simulink model "ThreeMotorModelSimulationXwithRangles"  (R2020b)
settings: Solver=ode14x  StartTime=0.0  StopTime=SimTime  FixedStep=SimStepTime  RelTol=1e-3
InitFcn:
  | StartupScript
StartFcn:
  | StartupScript
values from neighbouring files (symbols this model uses):
  CF = 372.0    (= 372)    [StartupScript.m]
  d2r = pi/180    (= 0.0174532925199)    [StartupScript.m]
  Isat = 10.0    (= 10)    [StartupScript.m]
  Ka = 1    [StartupScript.m]
  Kb = 1    [StartupScript.m]
  Kda = 50    [StartupScript.m]
  Kdb = 280    [StartupScript.m]
  Kdr = 3.4    [StartupScript.m]
  Kia = 150    [StartupScript.m]
  Kib = 200    [StartupScript.m]
  Kir = 6.1    [StartupScript.m]
  Kma = 19.5*1e-3    (= 0.0195)    [StartupScript.m]
  Kmb = 23.4*1e-3    (= 0.0234)    [StartupScript.m]
  Kmr = 29.9*1e-3    (= 0.0299)    [StartupScript.m]
  Kpa = 1250    [StartupScript.m]
  Kpb = 1500    [StartupScript.m]
  Kpr = 40    [StartupScript.m]
  Kr = 1    [StartupScript.m]
  PidLim = 1024    [StartupScript.m]
  PidUCGain = 5/1024    (= 0.0048828125)    [StartupScript.m]
  r2d = 180/pi    (= 57.2957795131)    [StartupScript.m]
  sensorGain = 1/1024.0    (= 0.0009765625)    [StartupScript.m]
  SimStepTime = 1e-3    (= 0.001)    [StartupScript.m]
  Vsat = 24.0    (= 24)    [StartupScript.m]
libraries: cstblocks x9, simulink x1
settings Model: Creator=nisch  LastModifiedBy=nisch

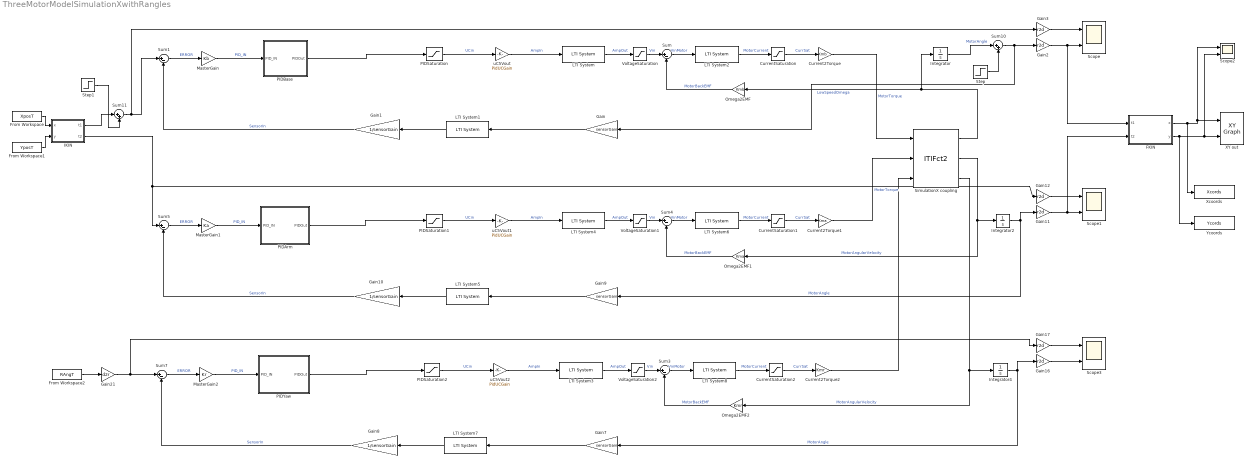
== system ThreeMotorModelSimulationXwithRangles ==
  Current2Torque : Gain  Gain=Kmb
  Current2Torque1 : Gain  Gain=Kma
  Current2Torque2 : Gain  Gain=Kmr
  CurrentSaturation : Saturate  UpperLimit=Isat  LowerLimit=-Isat
  CurrentSaturation1 : Saturate  UpperLimit=Isat  LowerLimit=-Isat
  CurrentSaturation2 : Saturate  UpperLimit=Isat  LowerLimit=-Isat
  FKIN : MATLAB Function  TreatAsAtomicUnit=on
  From Workspace : FromWorkspace  VariableName=XposT
  From Workspace1 : FromWorkspace  VariableName=YposT
  From Workspace2 : FromWorkspace  VariableName=RAngT  SampleTime=-1
  Gain : Gain  Gain=sensorGain
  Gain1 : Gain  Gain=1/sensorGain
  Gain10 : Gain  Gain=1/sensorGain
  Gain{2..3,11..12,16..17} (6 alike) : Gain  Gain=r2d
  Gain21 : Gain  Gain=d2r
  Gain7 : Gain  Gain=sensorGain
  Gain8 : Gain  Gain=1/sensorGain
  Gain9 : Gain  Gain=sensorGain
  IKIN : MATLAB Function  TreatAsAtomicUnit=on
  Integrator : Integrator
  Integrator2 : Integrator
  Integrator4 : Integrator
  LTI System : cstblocks/LTI System  sys=VoltageAmplifier  IC=[]
  LTI System1 : cstblocks/LTI System  sys=Hs  IC=[]
  LTI System2 : cstblocks/LTI System  sys=Electricalb  IC=[]
  LTI System3 : cstblocks/LTI System  sys=VoltageAmplifier  IC=[]
  LTI System4 : cstblocks/LTI System  sys=VoltageAmplifier  IC=[]
  LTI System5 : cstblocks/LTI System  sys=Hs  IC=[]
  LTI System6 : cstblocks/LTI System  sys=Electricala  IC=[]
  LTI System7 : cstblocks/LTI System  sys=Hs  IC=[]
  LTI System8 : cstblocks/LTI System  sys=Electricalr  IC=[]
  MasterGain : Gain  Gain=Kb
  MasterGain1 : Gain  Gain=Ka
  MasterGain2 : Gain  Gain=Kr
  Omega2EMF : Gain  Gain=Kmb
  Omega2EMF1 : Gain  Gain=Kma
  Omega2EMF2 : Gain  Gain=Kmr
  PIDArm : Subsystem
      mask Display: image('MATLABFcn.png'); % Use "Edit Image" on toolstrip to change.
  PIDBase : Subsystem
      mask Display: image('MATLABFcn.png'); % Use "Edit Image" on toolstrip to change.
  PIDSaturation : Saturate  UpperLimit=PidLim  LowerLimit=-PidLim
  PIDSaturation1 : Saturate  UpperLimit=PidLim  LowerLimit=-PidLim
  PIDSaturation2 : Saturate  UpperLimit=PidLim  LowerLimit=-PidLim
  PIDYaw : Subsystem
      mask Display: image('MATLABFcn.png'); % Use "Edit Image" on toolstrip to change.
  Scope{,1..3} (4 alike) : Scope  NumInputPorts=2
  SimulationX coupling : S-Function  FunctionName=ITIFct2  Parameters=ip, port, ts, nIn, nOut  SFunctionDeploymentMode=off  EnableBusSupport=off  mask{ip='localhost', port=4097, ts=SimStepTime, nIn=3, nOut=3}
      mask prompts: ip "Address: ip"; port "Port Number: port [-]"; ts "Communication Step Size: ts [s]"; nIn "Input Vector Dimension (to SimulationX): nIn [-]"; nOut "Output Vector Dimension (from SimulationX): nOut [-]"
      mask help: Coupling Element
  Step : Step  Time=0  After=30*d2r  SampleTime=0
  Step1 : Step  Time=0  After=0*d2r  SampleTime=0
  Sum{,1,3..5,7} (6 alike) : Sum  Inputs=|+-
  Sum10 : Sum  Inputs=|++
  Sum11 : Sum  Inputs=|++
  VoltageSaturation : Saturate  UpperLimit=Vsat  LowerLimit=-Vsat
  VoltageSaturation1 : Saturate  UpperLimit=Vsat  LowerLimit=-Vsat
  VoltageSaturation2 : Saturate  UpperLimit=Vsat  LowerLimit=-Vsat
  XY out : simulink/Sinks/XY Graph  xmin=-50  xmax=50  ymin=-50  ymax=50  st=-1
  Xcoords : ToWorkspace  VariableName=Xcords  SaveFormat=Timeseries  SampleTime=-1
  Ycoords : ToWorkspace  VariableName=Ycords  SaveFormat=Timeseries  SampleTime=-1
  uC5Vout : Gain  Gain=PidUCGain
  uC5Vout1 : Gain  Gain=PidUCGain
  uC5Vout2 : Gain  Gain=PidUCGain
  wires:
  LTI System/1 -> VoltageSaturation/1  "AmpOut"
  PIDSaturation/1 -> uC5Vout/1  "UCin"
  VoltageSaturation/1 -> Sum/1  "Vin"
  uC5Vout/1 -> LTI System/1  "AmpIn"
  Sum1/1 -> MasterGain/1  "ERROR"
  LTI System2/1 -> CurrentSaturation/1  "MotorCurrent"
  CurrentSaturation/1 -> Current2Torque/1  "CurrSat"
  Gain2/1 -> FKIN/1(t1), Scope/2
  Sum/1 -> LTI System2/1  "VinMotor"
  Omega2EMF/1 -> Sum/2  "MotorBackEMF"
  LTI System1/1 -> Gain1/1
  Gain1/1 -> Sum1/2  "SensorIn"
  Gain3/1 -> Scope/1
  Gain11/1 -> Scope1/2, FKIN/2(t2)
  IKIN/2(t2) -> Sum5/1, Gain12/1
  VoltageSaturation1/1 -> Sum4/1  "Vin"
  PIDSaturation1/1 -> uC5Vout1/1  "UCin"
  LTI System5/1 -> Gain10/1
  LTI System4/1 -> VoltageSaturation1/1  "AmpOut"
  SimulationX coupling/2 -> Omega2EMF1/1, Integrator2/1  "MotorAngularVelocity"
  LTI System6/1 -> CurrentSaturation1/1  "MotorCurrent"
  CurrentSaturation1/1 -> Current2Torque1/1  "CurrSat"
  Omega2EMF1/1 -> Sum4/2  "MotorBackEMF"
  uC5Vout1/1 -> LTI System4/1  "AmpIn"
  Sum4/1 -> LTI System6/1  "VinMotor"
  Integrator2/1 -> Gain11/1, Gain9/1  "MotorAngle"
  Gain12/1 -> Scope1/1
  Sum5/1 -> MasterGain1/1  "ERROR"
  Gain10/1 -> Sum5/2  "SensorIn"
  FKIN/1(x) -> Xcoords/1, XY out/1, Scope2/1
  FKIN/2(y) -> XY out/2, Scope2/2, Ycoords/1
  SimulationX coupling/1 -> Omega2EMF/1, Integrator/1  "LowSpeedOmega"
  Current2Torque/1 -> SimulationX coupling/1  "MotorTorque"
  Current2Torque1/1 -> SimulationX coupling/2  "MotorTorque"
  From Workspace1/1 -> IKIN/2(y)
  From Workspace/1 -> IKIN/1(x)
  Gain17/1 -> Scope3/1
  uC5Vout2/1 -> LTI System3/1  "AmpIn"
  Omega2EMF2/1 -> Sum3/2  "MotorBackEMF"
  Sum3/1 -> LTI System8/1  "VinMotor"
  CurrentSaturation2/1 -> Current2Torque2/1  "CurrSat"
  LTI System8/1 -> CurrentSaturation2/1  "MotorCurrent"
  VoltageSaturation2/1 -> Sum3/1  "Vin"
  Gain8/1 -> Sum7/2  "SensorIn"
  PIDSaturation2/1 -> uC5Vout2/1  "UCin"
  LTI System7/1 -> Gain8/1
  LTI System3/1 -> VoltageSaturation2/1  "AmpOut"
  SimulationX coupling/3 -> Omega2EMF2/1, Integrator4/1  "MotorAngularVelocity"
  Sum7/1 -> MasterGain2/1  "ERROR"
  Gain16/1 -> Scope3/2
  Integrator4/1 -> Gain16/1, Gain7/1  "MotorAngle"
  Current2Torque2/1 -> SimulationX coupling/3
  Integrator/1 -> Sum10/1  "MotorAngle"
  Sum10/1 -> Gain/1, Gain2/1
  Step/1 -> Sum10/2
  IKIN/1(t1) -> Sum11/1
  Sum11/1 -> Sum1/1, Gain3/1
  Step1/1 -> Sum11/2
  From Workspace2/1 -> Gain21/1
  Gain21/1 -> Gain17/1, Sum7/1
  Gain7/1 -> LTI System7/1
  Gain9/1 -> LTI System5/1
  Gain/1 -> LTI System1/1
  MasterGain/1 -> PIDBase/1(PID_IN)  "PID_IN"
  PIDBase/1(PIDOut) -> PIDSaturation/1
  MasterGain1/1 -> PIDArm/1(PID_IN)  "PID_IN"
  PIDArm/1(PIDOut) -> PIDSaturation1/1
  MasterGain2/1 -> PIDYaw/1(PID_IN)  "PID_IN"
  PIDYaw/1(PIDOut) -> PIDSaturation2/1

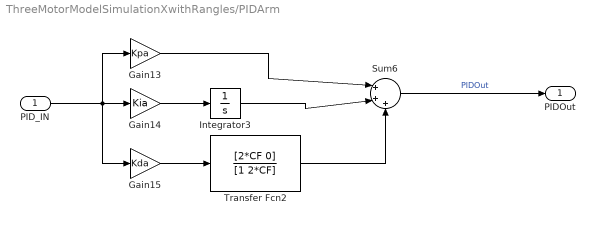
== system ThreeMotorModelSimulationXwithRangles/PIDArm ==
  PID_IN : Inport
  Gain13 : Gain  Gain=Kpa
  Gain14 : Gain  Gain=Kia
  Gain15 : Gain  Gain=Kda
  Integrator3 : Integrator
  Sum6 : Sum  Inputs=|+++
  Transfer Fcn2 : TransferFcn  Numerator=[2*CF 0]  Denominator=[1 2*CF]
  PIDOut : Outport
  wires:
  Integrator3/1 -> Sum6/2
  Gain13/1 -> Sum6/1
  Gain15/1 -> Transfer Fcn2/1
  PID_IN/1 -> Gain15/1, Gain14/1, Gain13/1
  Gain14/1 -> Integrator3/1
  Transfer Fcn2/1 -> Sum6/3
  Sum6/1 -> PIDOut/1  "PIDOut"

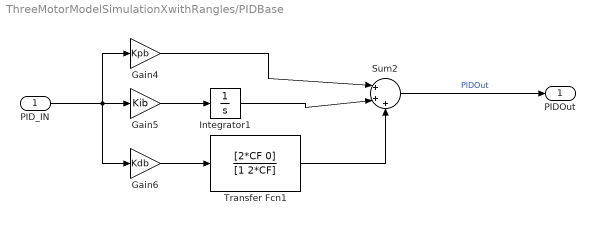
== system ThreeMotorModelSimulationXwithRangles/PIDBase ==
  PID_IN : Inport
  Gain4 : Gain  Gain=Kpb
  Gain5 : Gain  Gain=Kib
  Gain6 : Gain  Gain=Kdb
  Integrator1 : Integrator
  Sum2 : Sum  Inputs=|+++
  Transfer Fcn1 : TransferFcn  Numerator=[2*CF 0]  Denominator=[1 2*CF]
  PIDOut : Outport
  wires:
  Transfer Fcn1/1 -> Sum2/3
  Gain6/1 -> Transfer Fcn1/1
  PID_IN/1 -> Gain6/1, Gain5/1, Gain4/1
  Integrator1/1 -> Sum2/2
  Gain4/1 -> Sum2/1
  Gain5/1 -> Integrator1/1
  Sum2/1 -> PIDOut/1  "PIDOut"

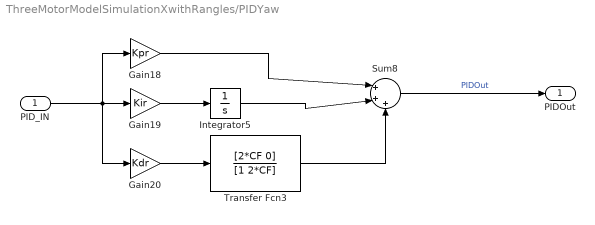
== system ThreeMotorModelSimulationXwithRangles/PIDYaw ==
  PID_IN : Inport
  Gain18 : Gain  Gain=Kpr
  Gain19 : Gain  Gain=Kir
  Gain20 : Gain  Gain=Kdr
  Integrator5 : Integrator
  Sum8 : Sum  Inputs=|+++
  Transfer Fcn3 : TransferFcn  Numerator=[2*CF 0]  Denominator=[1 2*CF]
  PIDOut : Outport
  wires:
  Integrator5/1 -> Sum8/2
  PID_IN/1 -> Gain20/1, Gain19/1, Gain18/1
  Transfer Fcn3/1 -> Sum8/3
  Gain20/1 -> Transfer Fcn3/1
  Gain19/1 -> Integrator5/1
  Gain18/1 -> Sum8/1
  Sum8/1 -> PIDOut/1  "PIDOut"

== matlab function ThreeMotorModelSimulationXwithRangles/IKIN ==
  data: x input; t1 output; y input; t2 output
function [t1, t2] = InverseKin(x, y)
    L1 = 30;
    L2 = 15;
    L3 = sqrt(x^2 + y^2);
    
    a = acos(complex((L1^2 + L3^2 - L2^2)/(2*L1*L3)));
    b = acos(complex((L1^2 + L2^2 - L3^2)/(2*L2*L1)));
    
    Theta = atan2(y,x);
    
    t1 = real((Theta + a));
    t2 = -real(pi-b); 
end

== matlab function ThreeMotorModelSimulationXwithRangles/FKIN ==
  data: t1 input; x output; t2 input; y output
function [x, y] = ForwardKin(t1, t2)
    
    Larm1 = 30;
    Larm2 = 15;
    
    arm1X = Larm1 * cos(t1*pi/180);
    arm1Y = Larm1 * sin(t1*pi/180);

    arm2X = Larm2 * cos((t2+t1)*pi/180) + arm1X;
    arm2Y = Larm2 * sin((t2+t1)*pi/180) + arm1Y;
    
    y = arm2Y;
    x = arm2X;
end
